simulink library "AeroActuators"  (R2025a)
settings: Solver=VariableStepAuto  StartTime=0.0  StopTime=10.0  RelTol=1e-3
undefined symbols (not defined in the file): act
settings Model: Creator=ASUS  LastModifiedBy=ASUS

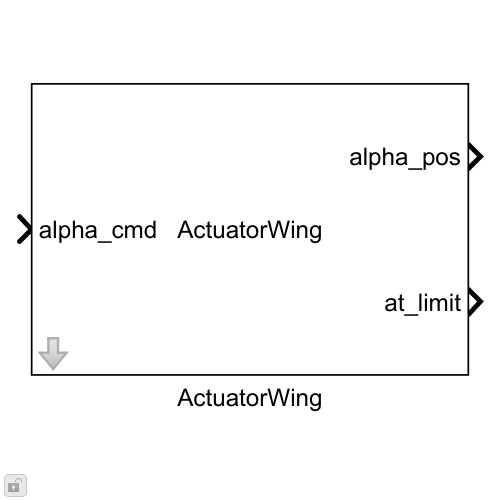
[thumbnail: Simulink's stored preview of the top-level diagram]
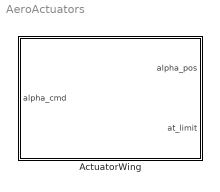
== system AeroActuators ==
  ActuatorWing : Subsystem  mask(Wing Actuator (RT)){tau=act.tau, Ts=0.001, rateLim=act.rateLim, clamp2=act.rwClamp, alpha0=0, limTol=1e-6}
      mask prompts: tau "Lag time constant tau [s]"; Ts "Discrete sample time Ts [s]"; rateLim "Slew-rate limit [deg/s]"; clamp2 "Angle clamp [lo hi] [deg]"; alpha0 "Initial angle alpha0 [deg]"; limTol "at_limit detection tolerance [deg]"
      mask help:
      | Discrete real-time wing-actuator model: command clamp -> first-order lag -> slew-rate limit
      | -> angle clamp.
      |
      | CHAIN (in this order, matching the offline solver's actuator envelope):
      |   alpha_cmd -> CmdClamp        clamp2 = [lo hi] [deg]   (see ANTI-WINDUP below)
      |             -> 1st-order lag   y[k] = a*y[k-1] + (1-a)*u[k],  a = exp(-Ts/tau)  (Unit Delay form)
      |             -> Rate Limiter    +/- rateLim [deg/s]
      |             -> Saturation      clamp2 = [lo hi] [deg]
      |             -> alpha_pos
      |
      | ANTI-WINDUP -- why the command is clamped at the INPUT as well as the output:
      |   The Rate Limiter's state is its own output, which sits BEFORE the output Saturation and is
      |   therefore not bounded by it. Fed a command beyond the mechanical range, that state ramps on
      |   past the end stop while alpha_pos sits still at the clamp, and on reversal the actuator must
      |   first unwind the excess before it moves - measured 1.6 s of phantom dead time for a +40 deg
      |   over-demand against the front-wing clamp [-25 0] (gate section D). A real actuator resting on
      |   an end stop reverses immediately. Clamping alpha_cmd first keeps the lag output, and hence the
      |   Rate Limiter state, inside [lo hi] at all times, which removes the windup without altering the
      |   mandated lag -> rate -> clamp order. For any command already inside clamp2 -- which is every
      |   command the ARFWr ECU issues, its stations being the clamp edges themselves - CmdClamp is a
      |   pass-through and the block is bit-identical to the un-clamped chain. The output Saturation is
      |   kept as the guard for the one remaining path to an out-of-range position, alpha0 set outside
      |   clamp2.
      |
      | OUTPUT 2, at_limit (boolean), is the OR of two simple detectors:
      |   (a) rate-saturated : |lagOut - rateLimOut| > limTol, i.e. the Rate Limiter actually clipped
      |       this step. Measured across the Rate Limiter rather than as a slope of alpha_pos on
      |       purpose: once the position is on a clamp it stops moving, so a slope test on alpha_pos
      |       would read "not slewing" exactly when the actuator is hardest against its command.
      |   (b) at a clamp edge: min(|alpha_pos - clamp2(1)|, |alpha_pos - clamp2(2)|) < limTol. This is
      |       a POSITION test, not a "being pushed against the stop" test - sitting on an edge with a
      |       matching command also reads at_limit = true.
      | limTol is a detection tolerance only; it has no effect on alpha_pos.
      |
      | DEFAULTS bind to the base-workspace struct act (simulink/params/actuatorParams.m), loaded by
      | the ARFWr_RT project startup file simulink/startup/projStartup.m. Ts has no act field, so its
      | default is the 1 ms RT actuator rate literal; override per instance if the harness runs slower.
      | For a front-wing instance set clamp2 = act.fwClamp; the default is the rear wing, act.rwClamp.
      |
      | Gate: simulink/validation/validateActuatorRT.m
      mask Display:
      | disp('ActuatorWing');
      | port_label('input',1,'alpha_cmd');
      | port_label('output',1,'alpha_pos'); port_label('output',2,'at_limit');

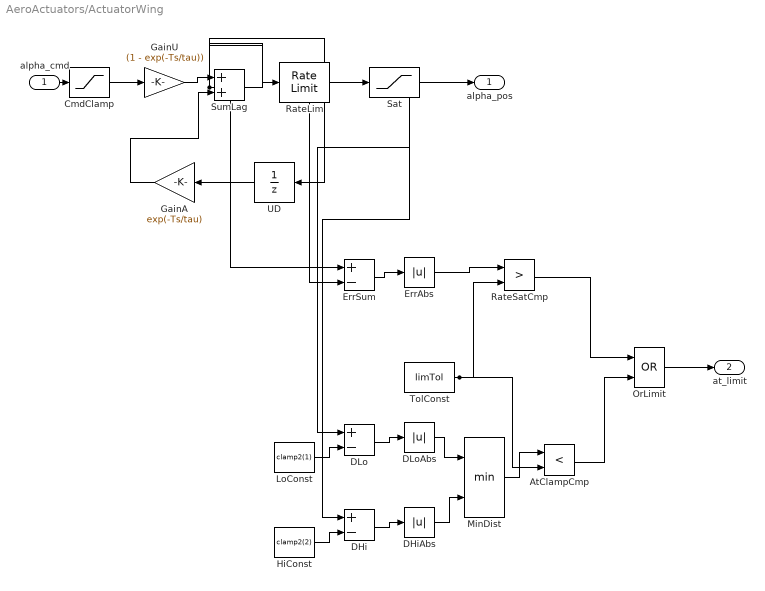
== system AeroActuators/ActuatorWing ==
  alpha_cmd : Inport
  AtClampCmp : RelationalOperator  Operator=<
  CmdClamp : Saturate  UpperLimit=clamp2(2)  LowerLimit=clamp2(1)
  DHi : Sum  Inputs=+-
  DHiAbs : Abs
  DLo : Sum  Inputs=+-
  DLoAbs : Abs
  ErrAbs : Abs
  ErrSum : Sum  Inputs=+-
  GainA : Gain  Gain=exp(-Ts/tau)
  GainU : Gain  Gain=(1 - exp(-Ts/tau))
  HiConst : Constant  Value=clamp2(2)
  LoConst : Constant  Value=clamp2(1)
  MinDist : MinMax  Inputs=2
  OrLimit : Logic  Operator=OR
  RateLim : RateLimiter  RisingSlewLimit=rateLim  FallingSlewLimit=-rateLim  SampleTimeMode=inherited  InitialCondition=alpha0
  RateSatCmp : RelationalOperator  Operator=>
  Sat : Saturate  UpperLimit=clamp2(2)  LowerLimit=clamp2(1)
  SumLag : Sum
  TolConst : Constant  Value=limTol
  UD : UnitDelay  InitialCondition=alpha0  SampleTime=Ts
  alpha_pos : Outport
  at_limit : Outport  Port=2
  wires:
  GainU/1 -> SumLag/1
  SumLag/1 -> RateLim/1, UD/1, ErrSum/1
  RateLim/1 -> Sat/1, ErrSum/2
  Sat/1 -> alpha_pos/1, DLo/1, DHi/1
  UD/1 -> GainA/1
  GainA/1 -> SumLag/2
  ErrSum/1 -> ErrAbs/1
  ErrAbs/1 -> RateSatCmp/1
  TolConst/1 -> RateSatCmp/2, AtClampCmp/2
  LoConst/1 -> DLo/2
  DLo/1 -> DLoAbs/1
  HiConst/1 -> DHi/2
  DHi/1 -> DHiAbs/1
  DLoAbs/1 -> MinDist/1
  DHiAbs/1 -> MinDist/2
  MinDist/1 -> AtClampCmp/1
  RateSatCmp/1 -> OrLimit/1
  AtClampCmp/1 -> OrLimit/2
  OrLimit/1 -> at_limit/1
  alpha_cmd/1 -> CmdClamp/1
  CmdClamp/1 -> GainU/1
